simulink model "NeuroFuzzyAfonso"  (R2019b)
settings: Solver=VariableStepAuto  StartTime=0.0  StopTime=100  RelTol=1e-3
libraries: fuzblock x1
settings Model: Creator=magnus  LastModifiedBy=Afonso

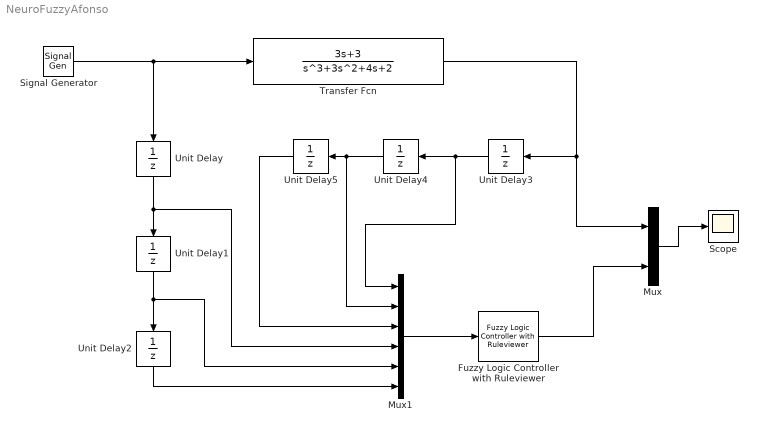
== system NeuroFuzzyAfonso ==
  Fuzzy Logic Controller with Ruleviewer : fuzblock/Fuzzy Logic  Controller  with Ruleviewer  fismatrix=FISFCMHyb  Ts=2
  Mux : Mux  Inputs=2
  Mux1 : Mux  Inputs=6
  Scope : Scope
  Signal Generator : SignalGenerator  Units=rad/sec
  Transfer Fcn : TransferFcn  Numerator=[3 3]  Denominator=[1 3 4 2]
  Unit Delay{,1..5} (6 alike) : UnitDelay  SampleTime=1/4  HasFrameUpgradeWarning=on
  wires:
  Signal Generator/1 -> Unit Delay/1, Transfer Fcn/1
  Transfer Fcn/1 -> Unit Delay3/1, Mux/1
  Mux/1 -> Scope/1
  Unit Delay/1 -> Unit Delay1/1, Mux1/4
  Unit Delay1/1 -> Unit Delay2/1, Mux1/5
  Mux1/1 -> Fuzzy Logic Controller with Ruleviewer/1
  Unit Delay3/1 -> Unit Delay4/1, Mux1/1
  Unit Delay4/1 -> Mux1/2, Unit Delay5/1
  Unit Delay5/1 -> Mux1/3
  Unit Delay2/1 -> Mux1/6
  Fuzzy Logic Controller with Ruleviewer/1 -> Mux/2
